simulink model "Prac3Simu"  (R2025a)
settings: Solver=ode45  StartTime=0.0  StopTime=10.0  MaxStep=0.01  RelTol=1e-3
InitFcn:
  | m1 = 290;
  | b1 = 1000;
  | m2 = 59;
  | k1 = 16182;
  | f = 0;
  | k2 = 19000;
undefined symbols (not defined in the file or in its folder): A1, w1

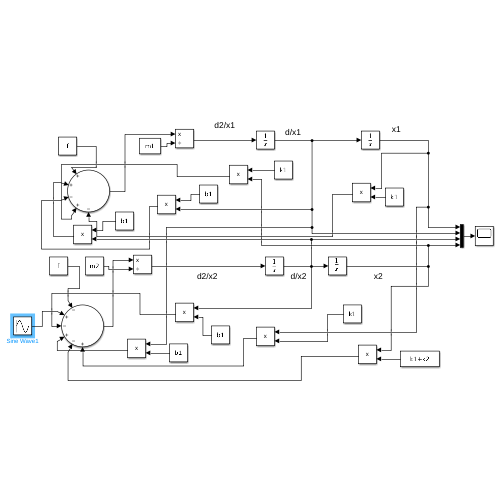
[thumbnail: Simulink's stored preview of the top-level diagram]
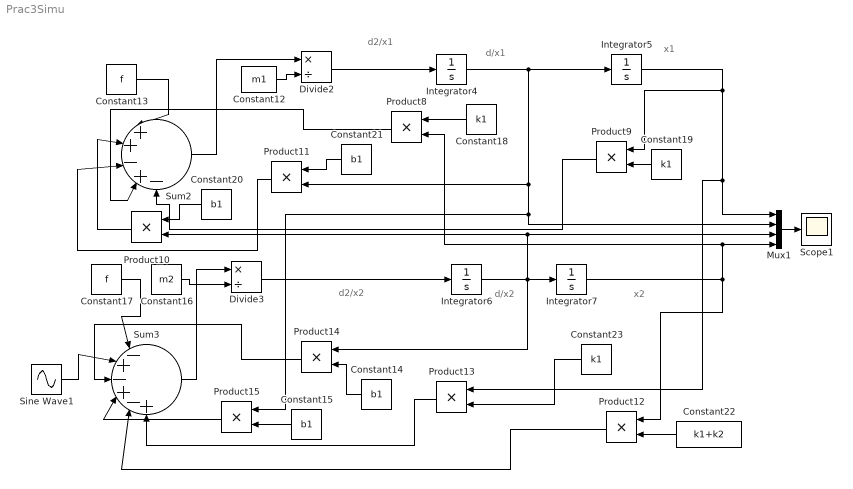
== system Prac3Simu ==
  note: x2
  note: d2/x2
  note: x1
  note: d2/x1
  note: d/x2
  note: d/x1
  Constant12 : Constant  Value=m1
  Constant13 : Constant  Value=f
  Constant{14..15,20..21} (4 alike) : Constant  Value=b1
  Constant16 : Constant  Value=m2
  Constant17 : Constant  Value=f
  Constant18 : Constant  Value=k1
  Constant19 : Constant  Value=k1
  Constant22 : Constant  Value=k1+k2
  Constant23 : Constant  Value=k1
  Divide2 : Product  Inputs=*/
  Divide3 : Product  Inputs=*/
  Integrator{4..7} (4 alike) : Integrator
  Mux1 : Mux
  Product{8..15} (8 alike) : Product
  Scope1 : Scope
      settings: ActiveDisplayYMinimum=-2.51376436496257E-5  ActiveDisplayYMaximum=3.8648514231052569E-5
  Sine Wave1 : Sin  Amplitude=A1  Frequency=w1  SampleTime=0
  Sum2 : Sum  Inputs=|++-+-
  Sum3 : Sum  Inputs=|-+-+-+
  wires:
  Mux1/1 -> Scope1/1
  Constant18/1 -> Product8/1
  Integrator6/1 -> Product14/1, Integrator7/1, Product10/2, Mux1/3
  Integrator5/1 -> Product9/1, Product13/1, Mux1/1
  Sine Wave1/1 -> Sum3/2
  Constant17/1 -> Sum3/1
  Product11/1 -> Sum2/3
  Product12/1 -> Sum3/5
  Integrator7/1 -> Product12/1, Mux1/4, Product8/2
  Constant20/1 -> Product10/1
  Constant16/1 -> Divide3/2
  Divide2/1 -> Integrator4/1
  Product8/1 -> Sum2/4
  Product15/1 -> Sum3/4
  Constant21/1 -> Product11/1
  Constant15/1 -> Product15/2
  Constant12/1 -> Divide2/2
  Constant13/1 -> Sum2/1
  Constant19/1 -> Product9/2
  Constant22/1 -> Product12/2
  Product9/1 -> Sum2/5
  Constant14/1 -> Product14/2
  Integrator4/1 -> Integrator5/1, Product15/1, Mux1/2, Product11/2
  Product14/1 -> Sum3/3
  Divide3/1 -> Integrator6/1
  Constant23/1 -> Product13/2
  Product10/1 -> Sum2/2
  Product13/1 -> Sum3/6
  Sum3/1 -> Divide3/1
  Sum2/1 -> Divide2/1
